simulink model "TestStandValidation"  (R2022b)
settings: Solver=ode14x  StartTime=0.0  StopTime=600  FixedStep=.5  RelTol=1e-3  AbsTol=1e-3  EnableMultiTasking=on
libraries: fl_lib x13, nesl_utility x8, sh_lib x3, simulink x2
settings Model: Creator=david  LastModifiedBy=david
settings SolverCC: AutoScaleAbsTol=off  AlgebraicLoopSolver=TrustRegion  PositivePriorityOrder=on  MaxZcPerStep=1
settings OptimizationCC: EnhancedBackFolding=on  PassReuseOutputArgsAs=Individual arguments  ZeroExternalMemoryAtStartup=off  ZeroInternalMemoryAtStartup=off  MaxStackSize=64  OptimizeBlockOrder=speed  DifferentSizesBufferReuse=on  OptimizationCustomize=off  EfficientTunableParamExpr=on
settings DebuggingCC: ParameterTunabilityLossMsg=error  UnconnectedInputMsg=warning  UnconnectedOutputMsg=warning  UnconnectedLineMsg=warning  SymbolicDimsDataTypeCodeGenerationDiagnostic=none  SFMachineParentedDataDiag=warning
settings HardwareCC: ProdBitPerPointer=32  ProdBitPerSizeT=32  ProdBitPerPtrDiffT=32  ProdLargestAtomicInteger=Long  ProdLargestAtomicFloat=Double  ProdWordSize=32  ProdLongLongMode=on  ProdHWDeviceType=ARM Compatible->ARM Cortex
settings ModelReferenceCC: EnableRefExpFcnMdlSchedulingChecks=on
settings SFSimCC: CustomCodeUndefinedFunction=UseInterfaceOnly
settings RTWCC: Description=Embedded Coder  SystemTargetFile=ert.tlc  HardwareBoard=Raspberry Pi  TLCOptions="-aInlineSetEventsForThisBaseRateFcn=TLC_FALSE -aSuppressMultiTaskScheduler=TLC_FALSE  -aRateBasedStepFcn=0"  TemplateMakefile=ert_default_tmf  Toolchain=GNU GCC Embedded Linux  BuildConfiguration=Faster Runs  DLArmComputeVersion=19.05
settings CodeAppCC: ForceParamTrailComments=on  IgnoreCustomStorageClasses=off  OperatorAnnotations=on  SimulinkDataObjDesc=on  SFDataObjDesc=on  InsertBlockDesc=on
settings ERTTargetCC: SupportVariableSizeSignals=on  ExtModeTransport=2  ExtModeStaticAlloc=on  ExtModeMexFile=ext_xcp  ExtModeIntrfLevel=Level2 - Open
settings SimscapeCC: SimscapeLogType=all  SimscapeLogSimulationStatistics=on  SimscapeLogDataHistory=10000

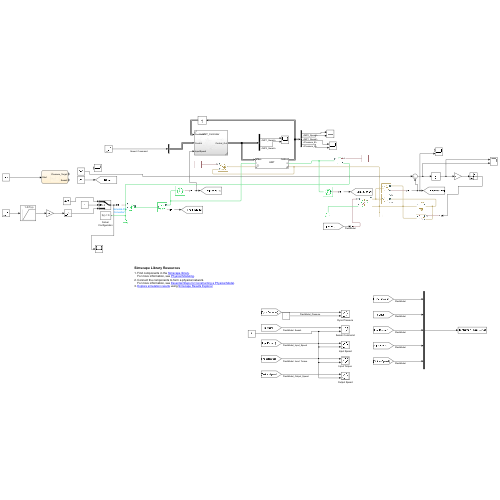
[thumbnail: Simulink's stored preview of the top-level diagram]
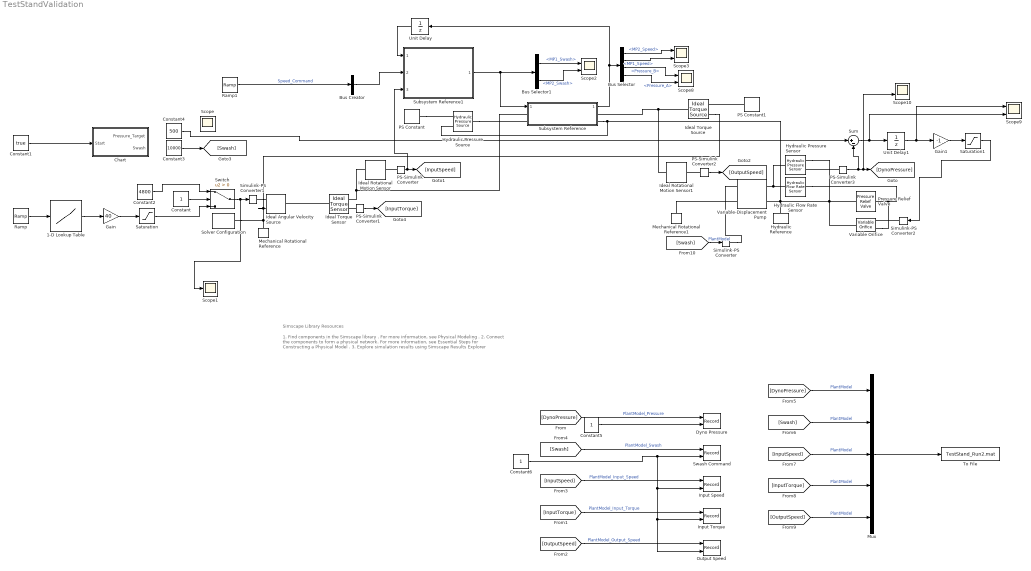
== system TestStandValidation ==
  note: 1. Find components in the Simscape library .
      | For more information, see Physical Modeling .
      | 2. Connect the components to form a physical network.
      | For more information, see Essential Steps for Constructing a Physical Model .
      | 3. Explore simulation results using Simscape Results Explorer
  note: Simscape Library Resources
  1-D Lookup Table : Lookup_n-D  NumberOfTableDimensions=1  BreakpointsForDimension1=[0,100,200]  Table=[0,100,100]  InternalRulePriority=Speed  RndMeth=Simplest
  Bus Creator : BusCreator  Inputs=1
  Bus Selector : BusSelector  OutputSignals=MP2_Speed,MP1_Speed,Pressure_B,Pressure_A
  Bus Selector1 : BusSelector  OutputSignals=MP1_Swash,MP2_Swash
  Chart : Stateflow chart  TreatAsAtomicUnit=on
  Constant : Constant
  Constant1 : Constant  Value=true
  Constant2 : Constant  Value=4800
  Constant3 : Constant  Value=10000
  Constant4 : Constant  Value=500
  Constant5 : Constant
  Constant6 : Constant
  Dyno Pressure : Record  FileSettingsInternal="{\"entries\":[{\"content\":{\"excelSettings\":{\"content\":{},\"type\":\"Streamout.ExcelSettings\"}},\"type\":\"Streamout.FileSettingStorage\",\"uuid\":\"fc692de2-203f-411b-8546-4268134a6f43\"}],\"packageUris\":[\"http://schema.mathworks.com/mf0/streamout_blocks/R2020a\"],\"version\":\"1.0\"}"  Layout=[1 1]  SignalsInternal="{\"entries\":[{\"content\":{\"signals\":[{\"content\":{\"blockPath\":[\"TestStandValidation/Dyno Pressure\"],\"channel\":[],\"dimensions\":[1,1],\"domain\":\"TestStandValidation/Dyno Pressure\",\"lineColor\":\"#77ac30\",\"plots\":[],\"port\":1,\"sid\":[\"\"],\"signalID\":5892,\"signalName\":\"PlantModel_Pressure\"},\"type\":\"RecordBlkView.Signal\",\"uuid\":\"6759c876-4caf-47ab-8fa9-06b73ff37c13\"},{\"content\":{\"blockPath\":[\"TestStandValidation/Dyno Pressure\"],\"channel\":[],\"dimensions\":[1],\"domain\":\"TestStandValidation/Dyno Pressure\",\"lineColor\":\"#ff6929\",\"plots\":[],\"port\":2,\"sid\":[\"\"],\"signalID\":5908,\"signalName\":\"Constant5\"},\"type\":\"RecordBlkView.Signal\",\"uuid\":\"3dbac6f9-3b5f-4268-9a5e-112a39dd79de\"}]},\"type\":\"RecordBlkView.InputSignals\",\"uuid\":\"4871bf7a-f447-42f9-aa95-e68e8457261b\"}],\"packageUris\":[\"http://schema.mathworks.com/mf0/streamout_blocks/R2020a\"],\"version\":\"1.0\"}"  VisualizationBindings="{\"xyplotplugin\":{\"info\":[{\"series\":[],\"subplotID\":1}]}}"  CompatibilityTag=XY
  Gain : Gain  Gain=40
  Gain1 : Gain  Gain=-1
  Hydraulic Flow Rate Sensor : fl_lib/Hydraulic/Hydraulic Sensors/Hydraulic Flow Rate Sensor
  Hydraulic Pressure Sensor : fl_lib/Hydraulic/Hydraulic Sensors/Hydraulic Pressure Sensor
  Hydraulic Pressure Source : fl_lib/Hydraulic/Hydraulic Sources/Hydraulic Pressure Source
      settings: InternalSimscapePortConfiguration="{\"Bottom\":[],\"Left\":[{\"id\":\"P\",\"label\":\"P\",\"type\":\"foundation.hydraulic.hydraulic\"}],\"Right\":[{\"id\":\"S\",\"label\":\"S\",\"type\":\"input\"},{\"id\":\"T\",\"label\":\"T\",\"type\":\"foundation.hydraulic.hydraulic\"}],\"Top\":[]}"
  Hydraulic Reference : fl_lib/Hydraulic/Hydraulic Elements/Hydraulic Reference
  Ideal Angular Velocity Source : fl_lib/Mechanical/Mechanical Sources/Ideal Angular Velocity Source
  Ideal Rotational Motion Sensor : fl_lib/Mechanical/Mechanical Sensors/Ideal Rotational Motion Sensor  reference=foundation.enum.MeasurementReference.absolute  acceleration_port=false  velocity_port=true  position_port=false  wrap_angle=false  offset=0 rad
      settings: InternalSimscapePortConfiguration="{\"Bottom\":[],\"Left\":[{\"id\":\"R\",\"label\":\"R\",\"type\":\"foundation.mechanical.rotational.rotational\"}],\"Right\":[{\"id\":\"W\",\"label\":\"W\",\"type\":\"output\"}],\"Top\":[]}"
  Ideal Rotational Motion Sensor1 : fl_lib/Mechanical/Mechanical Sensors/Ideal Rotational Motion Sensor  reference=foundation.enum.MeasurementReference.absolute  acceleration_port=false  velocity_port=true  position_port=false  wrap_angle=false  offset=0 rad
      settings: InternalSimscapePortConfiguration="{\"Bottom\":[],\"Left\":[{\"id\":\"R\",\"label\":\"R\",\"type\":\"foundation.mechanical.rotational.rotational\"}],\"Right\":[{\"id\":\"W\",\"label\":\"W\",\"type\":\"output\"}],\"Top\":[]}"
  Ideal Torque Sensor : fl_lib/Mechanical/Mechanical Sensors/Ideal Torque Sensor
  Ideal Torque Source : fl_lib/Mechanical/Mechanical Sources/Ideal Torque Source
  Input Speed : Record  FileSettingsInternal="{\"entries\":[{\"content\":{\"excelSettings\":{\"content\":{},\"type\":\"Streamout.ExcelSettings\"}},\"type\":\"Streamout.FileSettingStorage\",\"uuid\":\"303e2b9c-d083-49aa-bc0a-e5d82d300f27\"}],\"packageUris\":[\"http://schema.mathworks.com/mf0/streamout_blocks/R2020a\"],\"version\":\"1.0\"}"  Layout=[1 1]  SignalsInternal="{\"entries\":[{\"content\":{\"signals\":[{\"content\":{\"blockPath\":[\"TestStandValidation/Input Speed\"],\"channel\":[],\"dimensions\":[1,1],\"domain\":\"TestStandValidation/Input Speed\",\"lineColor\":\"#4dbeee\",\"plots\":[],\"port\":1,\"sid\":[\"\"],\"signalID\":5896,\"signalName\":\"PlantModel_Input_Speed\"},\"type\":\"RecordBlkView.Signal\",\"uuid\":\"d4d051ac-98b8-43f6-ae2d-0a14aa829deb\"},{\"content\":{\"blockPath\":[\"TestStandValidation/Input Speed\"],\"channel\":[],\"dimensions\":[1],\"domain\":\"TestStandValidation/Input Speed\",\"lineColor\":\"#b746ff\",\"plots\":[],\"port\":2,\"sid\":[\"\"],\"signalID\":5912,\"signalName\":\"Constant6\"},\"type\":\"RecordBlkView.Signal\",\"uuid\":\"1dd6f4b1-0012-4a19-ac8f-720520f4c72f\"}]},\"type\":\"RecordBlkView.InputSignals\",\"uuid\":\"a9c1dbe5-30fd-45ae-be23-b8d710dd0d2e\"}],\"packageUris\":[\"http://schema.mathworks.com/mf0/streamout_blocks/R2020a\"],\"version\":\"1.0\"}"  VisualizationBindings="{\"xyplotplugin\":{\"info\":[{\"series\":[],\"subplotID\":1}]}}"  CompatibilityTag=XY
  Input Torque : Record  FileSettingsInternal="{\"entries\":[{\"content\":{\"excelSettings\":{\"content\":{},\"type\":\"Streamout.ExcelSettings\"}},\"type\":\"Streamout.FileSettingStorage\",\"uuid\":\"1520097a-1fc7-4290-84c9-872b36d014ee\"}],\"packageUris\":[\"http://schema.mathworks.com/mf0/streamout_blocks/R2020a\"],\"version\":\"1.0\"}"  Layout=[1 1]  SignalsInternal="{\"entries\":[{\"content\":{\"signals\":[{\"content\":{\"blockPath\":[\"TestStandValidation/Input Torque\"],\"channel\":[],\"dimensions\":[1,1],\"domain\":\"TestStandValidation/Input Torque\",\"lineColor\":\"#a2142f\",\"plots\":[],\"port\":1,\"sid\":[\"\"],\"signalID\":5900,\"signalName\":\"PlantModel_Input_Torque\"},\"type\":\"RecordBlkView.Signal\",\"uuid\":\"115cb12d-78e0-4795-87ea-86ce04c0c533\"},{\"content\":{\"blockPath\":[\"TestStandValidation/Input Torque\"],\"channel\":[],\"dimensions\":[1],\"domain\":\"TestStandValidation/Input Torque\",\"lineColor\":\"#64d413\",\"plots\":[],\"port\":2,\"sid\":[\"\"],\"signalID\":5916,\"signalName\":\"Constant6\"},\"type\":\"RecordBlkView.Signal\",\"uuid\":\"a29e4725-8b6a-43ec-891b-9a3a902adfd8\"}]},\"type\":\"RecordBlkView.InputSignals\",\"uuid\":\"fb4c773b-a736-4f05-91a3-af0b7ee24964\"}],\"packageUris\":[\"http://schema.mathworks.com/mf0/streamout_blocks/R2020a\"],\"version\":\"1.0\"}"  VisualizationBindings="{\"xyplotplugin\":{\"info\":[{\"series\":[],\"subplotID\":1}]}}"  CompatibilityTag=XY
  Mechanical Rotational Reference : fl_lib/Mechanical/Rotational Elements/Mechanical Rotational Reference
  Mechanical Rotational Reference1 : fl_lib/Mechanical/Rotational Elements/Mechanical Rotational Reference
  Mux : Mux  Inputs=5
  Output Speed : Record  FileSettingsInternal="{\"entries\":[{\"content\":{\"excelSettings\":{\"content\":{},\"type\":\"Streamout.ExcelSettings\"}},\"type\":\"Streamout.FileSettingStorage\",\"uuid\":\"48d08ee3-f018-4f59-883a-76403190ead1\"}],\"packageUris\":[\"http://schema.mathworks.com/mf0/streamout_blocks/R2020a\"],\"version\":\"1.0\"}"  Layout=[1 1]  SignalsInternal="{\"entries\":[{\"content\":{\"signals\":[{\"content\":{\"blockPath\":[\"TestStandValidation/Output Speed\"],\"channel\":[],\"dimensions\":[1,1],\"domain\":\"TestStandValidation/Output Speed\",\"lineColor\":\"#139fff\",\"plots\":[],\"port\":1,\"sid\":[\"\"],\"signalID\":5904,\"signalName\":\"PlantModel_Output_Speed\"},\"type\":\"RecordBlkView.Signal\",\"uuid\":\"99b036fa-661a-428a-87c6-854da57f12f3\"},{\"content\":{\"blockPath\":[\"TestStandValidation/Output Speed\"],\"channel\":[],\"dimensions\":[1],\"domain\":\"TestStandValidation/Output Speed\",\"lineColor\":\"#ff13a6\",\"plots\":[],\"port\":2,\"sid\":[\"\"],\"signalID\":5920,\"signalName\":\"Constant6\"},\"type\":\"RecordBlkView.Signal\",\"uuid\":\"62bdbcdf-7509-425a-80c6-aa9544c12170\"}]},\"type\":\"RecordBlkView.InputSignals\",\"uuid\":\"5b70f11c-f2a8-4f43-8a9f-2664695f7061\"}],\"packageUris\":[\"http://schema.mathworks.com/mf0/streamout_blocks/R2020a\"],\"version\":\"1.0\"}"  VisualizationBindings="{\"xyplotplugin\":{\"info\":[{\"series\":[],\"subplotID\":1}]}}"  CompatibilityTag=XY
  PS Constant : fl_lib/Physical Signals/Sources/PS Constant  constant=100 psi
  PS Constant1 : fl_lib/Physical Signals/Sources/PS Constant  constant=-40
  PS-Simulink Converter : nesl_utility/PS-Simulink Converter  PhysicalDomain=network_engine_domain  SubClassName=ps_output  LeftPortType=input  RightPortType=output  PseudoPeriodic=off  Frequencies=[]  VectorFormat=inherit  Unit=rpm  AffineConversion=off
  PS-Simulink Converter1 : nesl_utility/PS-Simulink Converter  PhysicalDomain=network_engine_domain  SubClassName=ps_output  LeftPortType=input  RightPortType=output  PseudoPeriodic=off  Frequencies=[]  VectorFormat=inherit  Unit=N*m  AffineConversion=off
  PS-Simulink Converter2 : nesl_utility/PS-Simulink Converter  PhysicalDomain=network_engine_domain  SubClassName=ps_output  LeftPortType=input  RightPortType=output  PseudoPeriodic=off  Frequencies=[]  VectorFormat=inherit  Unit=rpm  AffineConversion=off
  PS-Simulink Converter3 : nesl_utility/PS-Simulink Converter  PhysicalDomain=network_engine_domain  SubClassName=ps_output  LeftPortType=input  RightPortType=output  PseudoPeriodic=off  Frequencies=[]  VectorFormat=inherit  Unit=psi  AffineConversion=off
  Pressure Relief Valve : sh_lib/Valves/Pressure Control Valves/Pressure Relief Valve  valve_area_spec=1  p_diff_TLU=[30.15e5 : 15e3 : 31.35e5] Pa  area_TLU=[1 : 1 : 9] .* 1e-5 m^2  area_max=1 m^2  pres_set=4000 psi  reg_range=5e5 Pa  C_d=0.7  A_leak=1e-12 m^2  lam_spec=1  B_lam=0.999  Re_cr=12  dynamic=0  tau=0.1 s  area_init=1e-12 m^2
      settings: InternalSimscapePortConfiguration="{\"Bottom\":[],\"Left\":[{\"id\":\"A\",\"label\":\"A\",\"type\":\"foundation.hydraulic.hydraulic\"}],\"Right\":[{\"id\":\"B\",\"label\":\"B\",\"type\":\"foundation.hydraulic.hydraulic\"}],\"Top\":[]}"
  Ramp : simulink/Sources/Ramp  slope=1  start=0  InitialOutput=0
  Ramp1 : simulink/Sources/Ramp  slope=1  start=0  InitialOutput=0
  Saturation : Saturate  UpperLimit=4000  LowerLimit=0
  Saturation1 : Saturate  UpperLimit=10000  LowerLimit=0
  Scope : Scope
  Scope1 : Scope
  Scope{2..3,8..10} (5 alike) : Scope  NumInputPorts=2
  Simulink-PS Converter : nesl_utility/Simulink-PS Converter  PhysicalDomain=network_engine_domain  SubClassName=ps_input  LeftPortType=input  RightPortType=output  PseudoPeriodic=off  Frequencies=[]  NoiseDistribution=none  NoiseParameters=[]  Unit=mm  AffineConversion=off  FilteringAndDerivatives=provide  SimscapeFilterOrder=1  InputFilterTimeConstant=0.001  UdotUserProvided=0
  Simulink-PS Converter1 : nesl_utility/Simulink-PS Converter  PhysicalDomain=network_engine_domain  SubClassName=ps_input  LeftPortType=input  RightPortType=output  PseudoPeriodic=off  Frequencies=[]  NoiseDistribution=none  NoiseParameters=[]  Unit=rpm  AffineConversion=off  FilteringAndDerivatives=filter  SimscapeFilterOrder=1  InputFilterTimeConstant=0.001  UdotUserProvided=0
  Simulink-PS Converter2 : nesl_utility/Simulink-PS Converter  PhysicalDomain=network_engine_domain  SubClassName=ps_input  LeftPortType=input  RightPortType=output  PseudoPeriodic=off  Frequencies=[]  NoiseDistribution=none  NoiseParameters=[]  Unit=mm  AffineConversion=off  FilteringAndDerivatives=provide  SimscapeFilterOrder=1  InputFilterTimeConstant=0.001  UdotUserProvided=0
  Solver Configuration : nesl_utility/Solver Configuration  PhysicalDomain=network_engine_domain  SubClassName=solver  LeftPortType=input  RightPortType=generic  Tones=[]  Harmonics=[]  SimulateNoise=off  Profile=off  UseLocalSampling=off  EnableSwitchedLinearOptims=on  FrequencyDomain=off  UseCCode=off  RelTol=0.001  AbsTol=1e-06  MinStep=1e-09  ToWorkspace=off  RevertToSquareIcSolve=off  NumHomotopyIterations=100  PhasorMode=off  PhasorModeNumHarmonics=1  ConsistencySolver=NEWTON_XTOL_AFTER_FTOL  IndexReductionMethod=DerivativeReplacement  DoDC=off  ResidualTolerance=1e-09  ConsistencyTolSource=GLOBAL  ConsistencyAbsTol=0.001  ConsistencyRelTol=0.001  ConsistencyTolFactor=0.001  UseLocalSolver=off  LocalSolverChoice=NE_BACKWARD_EULER_ADVANCER  ResolveIndetEquations=on  FunctionEvalNumThread=1  LocalSolverSampleTime=0.001  DoFixedCost=off  MaxNonlinIter=3  MaxModeIter=2  ComputeImpulses=off  ImpulseIterations=2  LinearAlgebra=auto  LinearAlgebraNumThread=0  EquationFormulation=NE_TIME_EF  DelaysMemoryBudget=1024  AutomaticFiltering=on  FilteringTimeConstant=0.001  PartitionStorageMethod=AS_NEEDED  PartitionMemoryBudget=1024  PartitionMethod=ROBUST
  Subsystem Reference : Subsystem  ReferencedSubsystem=HMT
      settings: PortSchema="{\"entries\":[{\"content\":{\"sides\":[{\"content\":{\"connectorIds\":[\"In1\",\"RConn1\",\"LConn2\"]},\"type\":\"ConnectorPlacement.EquallySpacedRectSide\",\"uuid\":\"acf7ffaa-0e23-471b-b66c-6886140d72c0\"},{\"content\":{\"connectorIds\":[\"Out1\",\"LConn1\",\"RConn2\"],\"side\":\"RIGHT\"},\"type\":\"ConnectorPlacement.EquallySpacedRectSide\",\"uuid\":\"49b39fe4-8ee4-458b-ac52-36807f0d6951\"},{\"content\":{\"connectorIds\":[],\"side\":\"TOP\"},\"type\":\"ConnectorPlacement.EquallySpacedRectSide\",\"uuid\":\"54c97d89-30c5-49b0-8e8a-cbf45f516668\"}]},\"type\":\"ConnectorPlacement.EquallySpacedConnector\",\"uuid\":\"36ff146f-267d-46ec-a3b7-0be64e1fcdaa\"}],\"packageUris\":[\"http://schema.mathworks.com/mf0/Connector/R2020b\"],\"version\":\"1.0\"}"
  Subsystem Reference1 : Subsystem  ReferencedSubsystem=HMT_Controller
  Sum : Sum  Inputs=|+-
  Swash Command : Record  FileSettingsInternal="{\"entries\":[{\"content\":{\"excelSettings\":{\"content\":{},\"type\":\"Streamout.ExcelSettings\"}},\"type\":\"Streamout.FileSettingStorage\",\"uuid\":\"60495974-50b7-4ee4-abdf-4082c28f3dcf\"}],\"packageUris\":[\"http://schema.mathworks.com/mf0/streamout_blocks/R2020a\"],\"version\":\"1.0\"}"  Layout=[1 1]  SignalsInternal="{\"entries\":[{\"content\":{\"signals\":[{\"content\":{\"blockPath\":[\"TestStandValidation/Swash Command\"],\"channel\":[],\"dimensions\":[1],\"domain\":\"TestStandValidation/Swash Command\",\"lineColor\":\"#fe330a\",\"plots\":[],\"port\":1,\"sid\":[\"\"],\"signalID\":5924,\"signalName\":\"PlantModel_Swash\"},\"type\":\"RecordBlkView.Signal\",\"uuid\":\"ebe939b5-06d7-4701-be7e-825b367b2817\"},{\"content\":{\"blockPath\":[\"TestStandValidation/Swash Command\"],\"channel\":[],\"dimensions\":[1],\"domain\":\"TestStandValidation/Swash Command\",\"lineColor\":\"#22b573\",\"plots\":[],\"port\":2,\"sid\":[\"\"],\"signalID\":5928,\"signalName\":\"Constant6\"},\"type\":\"RecordBlkView.Signal\",\"uuid\":\"a742e331-1927-4878-a4f2-9752a7ad0934\"}]},\"type\":\"RecordBlkView.InputSignals\",\"uuid\":\"5b6ef72d-983c-4201-9543-e6c867a78338\"}],\"packageUris\":[\"http://schema.mathworks.com/mf0/streamout_blocks/R2020a\"],\"version\":\"1.0\"}"  VisualizationBindings="{\"xyplotplugin\":{\"info\":[{\"series\":[],\"subplotID\":1}]}}"  CompatibilityTag=XY
  Switch : Switch  Criteria=u2 > Threshold  SaturateOnIntegerOverflow=off  InputSameDT=off
  To File : ToFile  Filename=TestStand_Run2.mat  SaveFormat=Timeseries
  Unit Delay : UnitDelay  SampleTime=-1  HasFrameUpgradeWarning=on
  Unit Delay1 : UnitDelay  SampleTime=-1  HasFrameUpgradeWarning=on
  Variable Orifice : sh_lib/Orifices/Variable Orifice  mdl_type=1  area_max=0.5 m^2  opening_max=10000 mm  opening_tab=[-.002, 0, .002, .005, .015] m  area_tab=[1e-09, 2.0352e-07, 4.0736e-05, .00011438, .00034356] m^2  pressure_tab=[-10000000, -5000000, -2000000, 2000000, 5000000, 10000000] Pa  flow_rate_tab=[-1e-07, -7.0711e-08, -4.4721e-08, 4.4721e-08, 7.0711e-08, 1e-07; -2.0352e-05, -1.4391e-05, -9.1017e-06, 9.1017e-06, 1.4391e-05, 2.0352e-05; -.0040736, -.0028805, -.0018218, .0018218, .0028805, .0040736; -.011438, -.0080879, -.0051152, .0051152, .0080879, .011438; -.034356, -.024293, -.015364, .015364, .024293, .034356] m^3/s  interp_method=1  extrap_method=1  or=1  C_d=0.7  x_0=0 m  A_leak=1e-12 m^2  lam_spec=1  B_lam=0.999  Re_cr=12  flow_rate_specify=off  flow_rate_priority=None  flow_rate=0 m^3/s  flow_rate_nominal_specify=off  flow_rate_nominal_unit=m^3/s  flow_rate_nominal_value=1  pressure_drop_specify=off  pressure_drop_priority=None  pressure_drop=0 Pa  pressure_drop_nominal_specify=off  pressure_drop_nominal_unit=Pa  pressure_drop_nominal_value=1
      settings: InternalSimscapePortConfiguration="{\"Bottom\":[],\"Left\":[{\"id\":\"S\",\"label\":\"S\",\"type\":\"input\"},{\"id\":\"A\",\"label\":\"A\",\"type\":\"foundation.hydraulic.hydraulic\"}],\"Right\":[{\"id\":\"B\",\"label\":\"B\",\"type\":\"foundation.hydraulic.hydraulic\"}],\"Top\":[]}"
  Variable-Displacement Pump : sh_lib/Pumps and Motors/Variable-Displacement Pump  mdl_type=1  stroke_max=10000 mm  D_max=5 in^3/rev  cntrl_mem_tab=[-.0075, -.0025, 0, .0025, .0075] m  displ_tab=[-30, -19, 0, 19, 30] cm^3/rev  interp_method=1  extrap_method=1  loss_spec=1  w_nominal=188 rad/s  pr_nominal=100e5 Pa  visc_nominal=18 cSt  dens_nominal=900 kg/m^3  efficiency_vol=0.92  no_load_torque=0.05 N*m  torque_pressure_coeff=0.6e-6 N*m/Pa  p_diff_eff_TLU=[100000, 1000000, 2000000] Pa  omega_eff_TLU=[25, 50, 100, 200, 300, 400] rad/s  displacement_eff_TLU=[-30, -19, 19, 30] cm^3/rev  vol_eff_TLU=repmat([.816, .908, .954, .977, .981, .984; .325, .663, .831, .916, .925, .946; .137, .568, .78, .892, .893, .91], 1, 1, 4)  mech_eff_TLU=repmat([.996, .996, .996, .996, .996, .996; .988, .989, .989, .989, .989, .99; .981, .981, .982, .982, .983, .984], 1, 1, 4)  p_diff_loss_TLU=[100000, 1000000, 2000000] Pa  omega_loss_TLU=[25, 50, 100, 200, 300, 400] rad/s  displacement_loss_TLU=[-30, -19, 19, 30] cm^3/rev  vol_loss_TLU=repmat([.023, .023, .023, .023, .0285, .032; .0844, .0842, .0845, .084, .1125, .108; .1079, .108, .11, .108, .1605, .18] * 1e-3, 1, 1, 4) m^3/s  mech_loss_TLU=repmat([.002, .002, .002, .002, .002, .002; .0607, .0556, .0556, .0556, .0556, .0505; .1937, .1937, .1833, .1833, .1729, .1626], 1, 1, 4) N*m  pressure_threshold=1e5 Pa  omega_threshold=10 rad/s  displacement_threshold=0.5 cm^3/rev  octant_check=0  pressure_check=0  min_valid_pressure=0 Pa  vol_eff_min=1e-3  vol_eff_max=1  mech_eff_min=1e-3  mech_eff_max=1
      settings: InternalSimscapePortConfiguration="{\"Bottom\":[],\"Left\":[{\"id\":\"C\",\"label\":\"C\",\"type\":\"input\"},{\"id\":\"S\",\"label\":\"S\",\"type\":\"foundation.mechanical.rotational.rotational\"}],\"Right\":[{\"id\":\"P\",\"label\":\"P\",\"type\":\"foundation.hydraulic.hydraulic\"},{\"id\":\"T\",\"label\":\"T\",\"type\":\"foundation.hydraulic.hydraulic\"}],\"Top\":[]}"
  wires:
  Switch/1 -> Scope1/1, Simulink-PS Converter1/1
  Constant/1 -> Switch/2
  Ramp/1 -> 1-D Lookup Table/1
  Saturation/1 -> Switch/3
  1-D Lookup Table/1 -> Gain/1
  Gain/1 -> Saturation/1
  Constant1/1 -> Chart/1(Start)
  Constant2/1 -> Switch/1
  PS-Simulink Converter3/1 -> Scope10/2, [DynoPressure], Sum/2
  Saturation1/1 -> Simulink-PS Converter2/1
  Sum/1 -> Unit Delay1/1, Scope9/2
  Gain1/1 -> Saturation1/1
  PS-Simulink Converter/1 -> Subsystem Reference1/3, [InputSpeed]
  PS-Simulink Converter2/1 -> [OutputSpeed]
  PS-Simulink Converter1/1 -> [InputTorque]
  [DynoPressure] -> Dyno Pressure/1  "PlantModel_Pressure"
  [InputTorque] -> Input Torque/1  "PlantModel_Input_Torque"
  [OutputSpeed] -> Output Speed/1  "PlantModel_Output_Speed"
  [InputSpeed] -> Input Speed/1  "PlantModel_Input_Speed"
  [Swash] -> Swash Command/1  "PlantModel_Swash"
  Mux/1 -> To File/1
  [DynoPressure] -> Mux/1  "PlantModel"
  [Swash] -> Mux/2  "PlantModel"
  [InputSpeed] -> Mux/3  "PlantModel"
  [InputTorque] -> Mux/4  "PlantModel"
  [OutputSpeed] -> Mux/5  "PlantModel"
  [Swash] -> Simulink-PS Converter/1  "PlantModel"
  Subsystem Reference1/1 -> Bus Selector1/1, Subsystem Reference/1
  Unit Delay/1 -> Subsystem Reference1/1
  Subsystem Reference/1 -> Unit Delay/1, Bus Selector/1
  Bus Creator/1 -> Subsystem Reference1/2
  Ramp1/1 -> Bus Creator/1  "Speed_Command"
  Bus Selector/2 -> Scope3/2  "<MP1_Speed>"
  Bus Selector/4 -> Scope8/2  "<Pressure_A>"
  Bus Selector/3 -> Scope8/1  "<Pressure_B>"
  Bus Selector/1 -> Scope3/1  "<MP2_Speed>"
  Constant3/1 -> [Swash]
  Constant4/1 -> Sum/1
  Constant5/1 -> Dyno Pressure/2
  Constant6/1 -> Output Speed/2, Input Torque/2, Input Speed/2, Swash Command/2
  Bus Selector1/1 -> Scope2/1  "<MP1_Swash>"
  Bus Selector1/2 -> Scope2/2  "<MP2_Swash>"
  Unit Delay1/1 -> Scope9/1, Gain1/1
  connections:
  Mechanical Rotational Reference/LConn1 -- Ideal Angular Velocity Source/RConn2 -- Ideal Torque Source/RConn2 -- Solver Configuration/RConn1
  Simulink-PS Converter1/RConn1 -- Ideal Angular Velocity Source/RConn1
  Ideal Torque Sensor/LConn1 -- Ideal Angular Velocity Source/LConn1
  Pressure Relief Valve/RConn1 -- Variable Orifice/RConn1 -- Hydraulic Pressure Sensor/RConn1 -- Hydraulic Pressure Source/RConn2 -- Subsystem Reference/RConn2 -- Variable-Displacement Pump/RConn2 -- Hydraulic Reference/LConn1
  Hydraulic Flow Rate Sensor/LConn1 -- Hydraulic Pressure Sensor/LConn1 -- Variable-Displacement Pump/RConn1
  Hydraulic Flow Rate Sensor/RConn2 -- Variable Orifice/LConn2 -- Pressure Relief Valve/LConn1
  PS-Simulink Converter1/LConn1 -- Ideal Torque Sensor/RConn2
  PS-Simulink Converter/LConn1 -- Ideal Rotational Motion Sensor/RConn1
  PS-Simulink Converter2/LConn1 -- Ideal Rotational Motion Sensor1/RConn1
  PS-Simulink Converter3/LConn1 -- Hydraulic Pressure Sensor/RConn2
  Simulink-PS Converter/RConn1 -- Variable-Displacement Pump/LConn1
  Simulink-PS Converter2/RConn1 -- Variable Orifice/LConn1
  Subsystem Reference/RConn1 -- Ideal Rotational Motion Sensor/LConn1 -- Ideal Torque Sensor/RConn1
  Hydraulic Pressure Source/LConn1 -- Subsystem Reference/LConn2
  PS Constant/RConn1 -- Hydraulic Pressure Source/RConn1
  Ideal Torque Source/LConn1 -- Ideal Rotational Motion Sensor1/LConn1 -- Subsystem Reference/LConn1
  PS Constant1/RConn1 -- Ideal Torque Source/RConn1
  Mechanical Rotational Reference1/LConn1 -- Variable-Displacement Pump/LConn2

== stateflow chart TestStandValidation/Chart ==
  state Wait
    en,du:
    Swash=0;
    Pressure_Target=0;
  state Constant_Speed
    en:
    Swash=0;
    state Constant_Swash
      en:
      Pressure_Target=0;
      state Waiting
      (default) -> Waiting
      (junction 13) -> Waiting : {Pressure_Target=Pressure_Target+50}
      (junction 11) -> (junction 13)
      Waiting -> (junction 11) : [after(500,msec)]
    (default) -> Constant_Swash
    (junction 18) -> Constant_Swash : {Swash=Swash+500}
    (junction 17) -> (junction 18)
    Constant_Swash -> (junction 16) : [Pressure_Target>=3000]
    (junction 16) -> (junction 17)
  (default) -> Wait
  Wait -> Constant_Speed : [Start]
  data: Start input; Pressure_Target output; Swash output
